simulink model "test"  (R2018a)
settings: Solver=VariableStepAuto  StartTime=0.0  StopTime=10.0  FixedStep=0.1  RelTol=1e-3
values from neighbouring files (symbols this model uses):
  g = 40    [params.m]
settings Model: Creator=soutrik  LastModifiedBy=soutrik

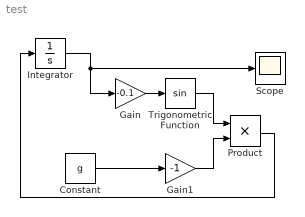
== system test ==
  Constant : Constant  Value=g
  Gain : Gain  Gain=-0.1
  Gain1 : Gain  Gain=-1
  Integrator : Integrator  InitialCondition=-1
  Product : Product
  Scope : Scope
  Trigonometric Function : Trigonometry
  wires:
  Gain1/1 -> Product/2
  Trigonometric Function/1 -> Product/1
  Gain/1 -> Trigonometric Function/1
  Integrator/1 -> Scope/1, Gain/1
  Product/1 -> Integrator/1
  Constant/1 -> Gain1/1
